simulink model "simu_MPC_diofant"  (R2023b)
settings: Solver=VariableStepAuto  StartTime=0.0  StopTime=12  RelTol=1e-3
values from neighbouring files (symbols this model uses):
  A = [-a_til(2:end)' [eye(length(a_til)-2); zeros(1,length(a_til)-2)]]    [MPC_deadtime.m]    (also in MPC_diofant.m = [1 -0.8]; SS_MPC_irrestrito.m = A'; SS_MPC_restrito.m = A')
  B = [b(2:end)']    [MPC_deadtime.m]    (also in MPC_diofant.m = [0.4 0.6]; SS_MPC_irrestrito.m = B'; SS_MPC_restrito.m = B')
  KF = K*F    [MPC_deadtime.m]    (also in MPC_diofant.m)
  KGp = [0 K*Gp]    [MPC_diofant.m]
  Kr = sum(K)    [MPC_SS.m]    (also in MPC_deadtime.m; MPC_diofant.m; MPC_ex1_c1.m; MPC_ex1_c2.m)
settings Model: Creator=sergio  LastModifiedBy=sergio

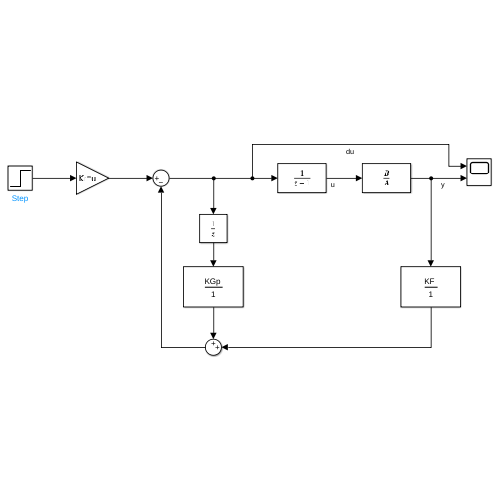
[thumbnail: Simulink's stored preview of the top-level diagram]
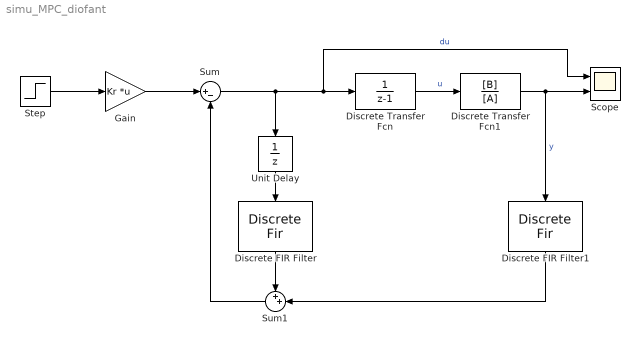
== system simu_MPC_diofant ==
  Discrete Transfer Fcn : DiscreteTransferFcn  Denominator=[1 -1]
  Discrete Transfer Fcn1 : DiscreteTransferFcn  Numerator=[B]  Denominator=[A]
  Discrete FIR Filter : DiscreteFir  Coefficients=[KGp]
  Discrete FIR Filter1 : DiscreteFir  Coefficients=[KF]
  Gain : Gain  Gain=Kr  Multiplication=Matrix(K*u)
  Scope : Scope  NumInputPorts=2
  Step : Step  Time=0  SampleTime=0
  Sum : Sum  Inputs=|+-
  Sum1 : Sum  Inputs=++|
  Unit Delay : UnitDelay  SampleTime=-1  HasFrameUpgradeWarning=on
  wires:
  Discrete Transfer Fcn/1 -> Discrete Transfer Fcn1/1  "u"
  Unit Delay/1 -> Discrete FIR Filter/1
  Sum1/1 -> Sum/2
  Gain/1 -> Sum/1
  Step/1 -> Gain/1
  Sum/1 -> Unit Delay/1, Discrete Transfer Fcn/1, Scope/1  "du"
  Discrete Transfer Fcn1/1 -> Scope/2, Discrete FIR Filter1/1  "y"
  Discrete FIR Filter1/1 -> Sum1/2
  Discrete FIR Filter/1 -> Sum1/1
